simulink model "BPSKDemodulation"  (R2019b)
settings: Solver=VariableStepAuto  StartTime=0.0  StopTime=10.0  RelTol=1e-3
libraries: dspfdesign x2, commchan3 x1, dspsigops x1, commsynccomp2 x1, commsink2 x1, commfilt2 x1
settings Model: Creator=z3454314  LastModifiedBy=z3454314

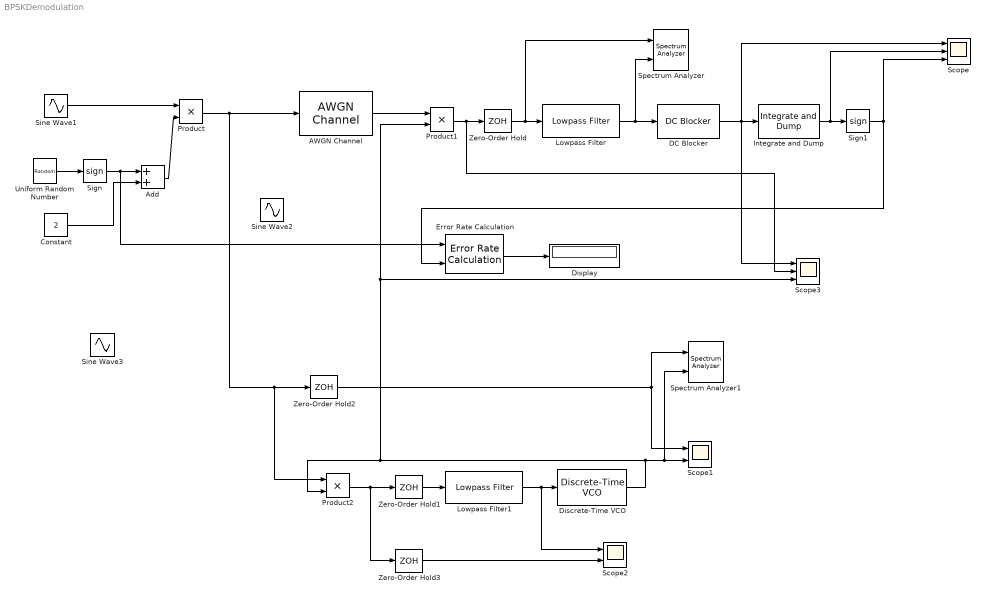
== system BPSKDemodulation ==
  AWGN Channel : commchan3/AWGN Channel  InputProcessing=Columns as channels (frame based)  seed=67  noiseMode="Signal to noise ratio  (SNR)"  EbNodB=30  EsNodB=10  SNRdB=50  bitsPerSym=1  Ps=0.5  Tsym=1/500  variance=1
      settings: SourceProductName=Communications Toolbox
  Add : Sum
  Constant : Constant  Value=2
  DC Blocker : dspsigops/DC Blocker  Algorithm=IIR  NormalizedBandwidth=0.001  Length=8  Order=6  SimulateUsing=Code generation
      settings: SourceProductName=DSP System Toolbox  SourceProductBaseCode=DS
  Discrete-Time VCO : commsynccomp2/Discrete-Time VCO  Ac=1  Fc=8000  Kc=100  Ph=0  ts=1/500e3
      settings: SourceProductName=Communications Toolbox  SourceProductBaseCode=CM
  Display : Display
  Error Rate Calculation : commsink2/Error Rate Calculation  N=2  st_delay=0  cp_mode=Entire frame  subframe=[]  PMode=Port  WsName=ErrorVec  RsMode2=off  stop=off  numErr=100  maxBits=1e6
      settings: SourceProductName=Communications Toolbox
  Integrate and Dump : commfilt2/Integrate and Dump  obssamples=500  offsetsamples=23  nodump=off  roundingMode=Floor  overflowMode=off  outputDataTypeStr=Inherit: Same as accumulator  outputLastDataTypeStr=Inherit: Same as accumulator
      settings: SourceProductName=Communications Toolbox
  Lowpass Filter : dspfdesign/Lowpass Filter  FilterType=FIR  DesignForMinimumOrder=on  FilterOrder=50  PassbandFrequency=6e3  StopbandFrequency=10e3  PassbandRipple=0.1  StopbandAttenuation=80  InheritSampleRate=on  SampleRate=44100  SimulateUsing=Interpreted execution  roundingMode=Floor  coeffsDataTypeStr=fixdt(1,16)
  Lowpass Filter1 : dspfdesign/Lowpass Filter  FilterType=FIR  DesignForMinimumOrder=on  FilterOrder=50  PassbandFrequency=5e3  StopbandFrequency=8e3  PassbandRipple=0.1  StopbandAttenuation=80  InheritSampleRate=on  SampleRate=500e3  SimulateUsing=Interpreted execution  roundingMode=Floor  coeffsDataTypeStr=fixdt(1,16)
  Product : Product
  Product1 : Product
  Product2 : Product
  Scope : Scope  NumInputPorts=3
  Scope1 : Scope  NumInputPorts=2
  Scope2 : Scope  NumInputPorts=2
  Scope3 : Scope  NumInputPorts=3
  Sign : Signum
  Sign1 : Signum
  Sine Wave1 : Sin  Frequency=8055*2*pi  SampleTime=0
  Sine Wave2 : Sin  Frequency=8000*2*pi  SampleTime=0
  Sine Wave3 : Sin  Frequency=8020*2*pi  SampleTime=0
  Spectrum Analyzer : SpectrumAnalyzer  NumInputPorts=2
  Spectrum Analyzer1 : SpectrumAnalyzer  NumInputPorts=2
  Uniform Random Number : UniformRandomNumber  SampleTime=1/1000
  Zero-Order Hold{,1..3} (4 alike) : ZeroOrderHold  SampleTime=1/500e3
  wires:
  Sine Wave1/1 -> Product/1
  Uniform Random Number/1 -> Sign/1
  Error Rate Calculation/1 -> Display/1
  Product/1 -> Product2/1, Zero-Order Hold2/1, AWGN Channel/1
  Zero-Order Hold/1 -> Spectrum Analyzer/1, Lowpass Filter/1
  Product1/1 -> Scope3/2, Zero-Order Hold/1
  AWGN Channel/1 -> Product1/1
  Integrate and Dump/1 -> Scope/2, Sign1/1
  Sign1/1 -> Scope/3, Error Rate Calculation/2
  Sign/1 -> Error Rate Calculation/1, Add/1
  Constant/1 -> Add/2
  Lowpass Filter/1 -> DC Blocker/1, Spectrum Analyzer/2
  Lowpass Filter1/1 -> Scope2/1, Discrete-Time VCO/1
  Product2/1 -> Zero-Order Hold3/1, Zero-Order Hold1/1
  Zero-Order Hold3/1 -> Scope2/2
  Zero-Order Hold2/1 -> Scope1/1, Spectrum Analyzer1/1
  Zero-Order Hold1/1 -> Lowpass Filter1/1
  Add/1 -> Product/2
  Discrete-Time VCO/1 -> Product1/2, Scope3/3, Product2/2, Spectrum Analyzer1/2, Scope1/2
  DC Blocker/1 -> Scope3/1, Scope/1, Integrate and Dump/1
